simulink model "testemplanner_cs"  (R2020a)
settings: Solver=ode5  StartTime=0.0  StopTime=24  FixedStep=1/1000  RelTol=1e-3
PreLoadFcn:
  | mbxruntime.callbacks.PreLoadFcn(bdroot);
PostLoadFcn:
  | mbxruntime.callbacks.PostLoadFcn(bdroot);
InitFcn:
  | mbxruntime.callbacks.InitFcn(bdroot);
StartFcn:
  | mbxruntime.callbacks.StartFcn(bdroot);
StopFcn:
  | mbxruntime.callbacks.StopFcn(bdroot);
model workspace (MAT data in the model file):
  mbox_table : object (value not decoded)
  model_closed = 0
  sim_status = 0
values from neighbouring files (symbols this model uses):
  c_factor = 43.75    [emplanner_init.m]
  cf = -175016    [emplanner_init.m]
  cr = -130634    [emplanner_init.m]
  global_path_x = [0.057304 1.05668625507 2.05480936558 3.05165624935 4.04722112279 5.04150235808 6.03449985569 7.02621407764 8.01664569183 9.00579544113 9.99366409523 10.9802524329 ... (3001 elements, 3001x1)]    [global_path.mat]
  global_path_y = [8.29 8.29 8.29 8.29 8.29 8.29 8.29 8.29 8.29 8.29 8.29 8.29 ... (3001 elements, 3001x1)]    [global_path.mat]
  KD_PID_distance = 0.0    (= 0)    [emplanner_init.m]
  KD_PID_speed = 0    [emplanner_init.m]
  KI_PID_distance = 0.0    (= 0)    [emplanner_init.m]
  KI_PID_speed = 0    [emplanner_init.m]
  KP_PID_distance = 0.5    [emplanner_init.m]
  KP_PID_speed = 1.8    [emplanner_init.m]
  la = 1.265    [emplanner_init.m]
  lb = 2.947-1.265    (= 1.682)    [emplanner_init.m]
  LQR_K1 = k(:,1)'    [emplanner_init.m]
  LQR_K2 = k(:,2)'    [emplanner_init.m]
  LQR_K3 = k(:,3)'    [emplanner_init.m]
  LQR_K4 = k(:,4)'    [emplanner_init.m]
  m = 2020    [emplanner_init.m]
  rack_displacement = [-39.14 , -37.2 , -35.29 , -33.43 , -31.6 , -29.81 , -28.06 , -26.34 , -24.66 ,      -23.01 , -21.38 , -19.79 , -18.23 , -16.69 , -15.18 , -13.7 , -12.23 , -10.8 , -9.38 , -7.98 ,     -6.61 , -5.25 , -3.91 , -2.59 , -1.29 , 0 , 1.27 , 2.54 , 3.78 , 5.02 , 6.24 , 7.46 , 8.66 ,      9.86 , 11.05 , 12.24 , 13.41 , 14.59 , 15.76 , 16.92 , 18.09 , 19.25 , 20.42 , 21.59 , 22.76 ,      23.93 , 25.11 , 26 ...(+26 chars)    [emplanner_init.m]
  right_wheel_ground = [-70 ,-67.2 , -64.4 , -61.6 , -58.8 , -56 , -53.2 , -50.4 , -47.6 , -44.8 , -42 ,      -39.2 , -36.4 , -33.6 , -30.8 , -28 , -25.2 , -22.4 , -19.6 , -16.8 , -14 , -11.2 , -8.4 , -5.6 ,      -2.8 , 0 , 2.8 , 5.6 , 8.4 , 11.2 , 14 , 16.8 , 19.6 , 22.4 , 25.2 , 28 , 30.8 , 33.6 , 36.4 ,      39.2 , 42 , 44.8 , 47.6 , 50.4 , 53.2 , 56 , 58.8 , 61.6 , 64.4 , 67.2 , 70 ]    [emplanner_init.m]
  vx_break_point = zeros(1,5000)    [emplanner_init.m]
undefined symbols (not defined in the file or in its folder): aubr, DiscIntNeverNeededParam, tablebr, vubr
libraries: PreScanSimulinkLibrary x9, Solver_SF x1, simulink_extras x1
(part 7 of 9)

== matlab function testemplanner_cs/Audi_A8_Sedan_1/decision&planning module/EM Planner/obs1/MATLAB Function2 ==
  data: x_set input; match_point_index_set output; y_set input; frenet_path_x input; frenet_path_y input; frenet_path_heading input; frenet_path_kappa input; proj_x_set output; proj_y_set output; proj_heading_set output; proj_kappa_set output
function [match_point_index_set,proj_x_set, proj_y_set,proj_heading_set,proj_kappa_set] = ...
    fcn(x_set,y_set,frenet_path_x,frenet_path_y,frenet_path_heading,frenet_path_kappa)
%该函数将批量计算x_set，y_set中的xy，在frenet_path下的投影的信息
%输入 x_set,y_set，待投影的点的集合
%x_set,y_set,frenet_path_x,frenet_path_y,frenet_path_heading,frenet_path_kappa
%曲线在直角坐标系下的x，y，heading，kappa
%输出：match_point_index_set 匹配点在frenet_path下的编号的集合(即从全局路径第一个点开始数，第几个点是匹配点)
%     proj_x y heading kappa 投影的x,y,heading,kappa的集合

% 由于事先不知道x_set中到底有多少个点需要投影，因此事先声明一个最大的数量的点作为缓冲
n = 128;
% 并且由于不知道投影点的个数，所以也不知道输出的个数，因此输出也要做缓冲，用nan表示不存在的点
% 输出最多输出128个
% 输出初始化
match_point_index_set = ones(n,1) * nan;
proj_x_set = ones(n,1) * nan;
proj_y_set = ones(n,1) * nan;
proj_heading_set = ones(n,1) * nan;
proj_kappa_set = ones(n,1) * nan;

%找匹配点，需要利用上一个周期的结果作为下一个周期遍历的起点，因此需要声明两个全局变量
persistent is_first_run;
persistent pre_match_point_index_set;
persistent pre_frenet_path_x;
persistent pre_frenet_path_y;
persistent pre_frenet_path_heading;
persistent pre_frenet_path_kappa;
%算法主函数入口

if isempty(is_first_run)
    %该if分支表示函数首次运行
    is_first_run = 0;
    pre_frenet_path_x = frenet_path_x;
    pre_frenet_path_y = frenet_path_y;
    pre_frenet_path_heading = frenet_path_heading;
    pre_frenet_path_kappa = frenet_path_kappa;
    %要记录首次运行计算的匹配点的结果供下个周期运行，先初始化
    pre_match_point_index_set = ones(n,1) * nan;
    %对x_set,y_set的点做遍历，找到他们的匹配点
    for i = 1 : length(x_set)
        if isnan(x_set(i))
            break;
        end
        %首次运行时，没有任何提示，只能从frenet path的第一个点开始找
        start_search_index = 1;
        % 声明increase_count，用于表示在遍历时distance连续增加的个数
        increase_count = 0;
        % 开始遍历
        min_distance = inf;
        for j = start_search_index : length(frenet_path_x)
            distance = (x_set(i) - frenet_path_x(j))^2 + (y_set(i) - frenet_path_y(j))^2;
            if distance < min_distance
                min_distance = distance;
                match_point_index_set(i) = j;
                increase_count = 0;
            else
                increase_count = increase_count + 1;
            end
            %如果distance连续增加50次就不要再遍历了，节省时间
            if increase_count > 50
                break;
            end
        end
        
        %如何通过匹配点计算投影点，请参见《自动驾驶控制算法第七讲》
        %或《自动驾驶决策规划算法》第一章第三节
        
        %取出匹配点的编号
        match_point_index = match_point_index_set(i);
        %取出匹配点的信息
        match_point_x = frenet_path_x(match_point_index);
        match_point_y = frenet_path_y(match_point_index);
        match_point_heading = frenet_path_heading(match_point_index);
        match_point_kappa = frenet_path_kappa(match_point_index);
        %计算匹配点的方向向量与法向量
        vector_match_point = [match_point_x;match_point_y];
        vector_match_point_direction = [cos(match_point_heading);sin(match_point_heading)];
        %声明待投影点的位矢
        vector_r = [x_set(i);y_set(i)];
        
       %通过匹配点计算投影点
       vector_d = vector_r - vector_match_point;
       ds = vector_d' * vector_match_point_direction;
       vector_proj_point = vector_match_point + ds * vector_match_point_direction;
       proj_heading = match_point_heading + match_point_kappa * ds;
       proj_kappa = match_point_kappa;
       %计算结果输出
       proj_x_set(i) = vector_proj_point(1);
       proj_y_set(i) = vector_proj_point(2);
       proj_heading_set(i) = proj_heading;
       proj_kappa_set(i) = proj_kappa;
    end
    %匹配点的计算结果保存，供下一个周期使用
    pre_match_point_index_set = match_point_index_set;
else
    %此if分支表示不是首次运行
    
    %对每个x_set上的点做处理
    for i = 1 : length(x_set)
        %不是首次运行，对于点x_set(i),y_set(i)来说,start_search_index =
        %pre_match_point_index_set(i)
        start_search_index = pre_match_point_index_set(i);%上个周期匹配点的编号作为本周期搜索的起点
        % 声明increase_count，用于表示在遍历时distance连续增加的个数
        %%%%%%%%%
        %对于障碍物检测而言，当感知第一次检测到障碍物时，算法并不是首次运行，此时 
        %pre_match_point_index_set的值是nan，如果还用上一时刻的结果作为本周期搜索的起点
        %必然会出问题，所以要修改
        % 声明increase_count_limit
        increase_count_limit = 5;
        if isnan(start_search_index)
            %没有上个周期的结果，那就不能只检查5次了
            increase_count_limit = 50;
            %搜索起点也要设为1
            start_search_index = 1;
        end
        increase_count = 0;
        % 开始遍历
        %这里多一个步骤，判断遍历的方向
        %计算上个周期匹配点的位矢
        vector_pre_match_point = [pre_frenet_path_x(start_search_index);pre_frenet_path_y(start_search_index)];
        vector_pre_match_point_direction = ...
            [cos(pre_frenet_path_heading(start_search_index));sin(pre_frenet_path_heading(start_search_index))];
        %判断遍历的方向
        flag = ([x_set(i);y_set(i)] - vector_pre_match_point)' * vector_pre_match_point_direction;
        min_distance = inf;
        if flag > 0.001
            for j = start_search_index : length(frenet_path_x)
                distance = (x_set(i) - frenet_path_x(j))^2 + (y_set(i) - frenet_path_y(j))^2;
                if distance < min_distance
                    min_distance = distance;
                    match_point_index_set(i) = j;
                    increase_count = 0;
                else
                    increase_count = increase_count + 1;
                end
                %如果distance连续增加increase_count_limit次就不要再遍历了，节省时间
                if increase_count > increase_count_limit
                    break;
                end
            end
        elseif flag < - 0.001
            for j = start_search_index : -1 : 1
                distance = (x_set(i) - frenet_path_x(j))^2 + (y_set(i) - frenet_path_y(j))^2;
                if distance < min_distance
                    min_distance = distance;
                    match_point_index_set(i) = j;
                    increase_count = 0;
                else
                    increase_count = increase_count + 1;
                end
                %如果distance连续增加increase_count_limit次就不要再遍历了，节省时间
                if increase_count > increase_count_limit
                    break;
                end
            end
        else
            match_point_index_set(i) = start_search_index;
        end
        
        %如何通过匹配点计算投影点，请参见《自动驾驶控制算法第七讲》
        %或《自动驾驶决策规划算法》第一章第三节
        
        %取出匹配点的编号
        match_point_index = match_point_index_set(i);
        %取出匹配点的信息
        match_point_x = frenet_path_x(match_point_index);
        match_point_y = frenet_path_y(match_point_index);
        match_point_heading = frenet_path_heading(match_point_index);
        match_point_kappa = frenet_path_kappa(match_point_index);
        %计算匹配点的方向向量与法向量
        vector_match_point = [match_point_x;match_point_y];
        vector_match_point_direction = [cos(match_point_heading);sin(match_point_heading)];
        %声明待投影点的位矢
        vector_r = [x_set(i);y_set(i)];
        
       %通过匹配点计算投影点
       vector_d = vector_r - vector_match_point;
       ds = vector_d' * vector_match_point_direction;
       vector_proj_point = vector_match_point + ds * vector_match_point_direction;
       proj_heading = match_point_heading + match_point_kappa * ds;
       proj_kappa = match_point_kappa;
       %计算结果输出
       proj_x_set(i) = vector_proj_point(1);
       proj_y_set(i) = vector_proj_point(2);
       proj_heading_set(i) = proj_heading;
       proj_kappa_set(i) = proj_kappa;
  
    end
    %匹配点的计算结果保存，供下一个周期使用
    pre_match_point_index_set = match_point_index_set;
    pre_frenet_path_x = frenet_path_x;
    pre_frenet_path_y = frenet_path_y;
    pre_frenet_path_heading = frenet_path_heading;
    pre_frenet_path_kappa = frenet_path_kappa;
end

== matlab function testemplanner_cs/Audi_A8_Sedan_1/decision&planning module/EM Planner/obs1/obs_fliter ==
  data: host_x input; obs_x_set_gcs_afterfliter output; host_y input; host_heading_xy input; obs_x_set_gcs input; obs_y_set_gcs input; obs_velocity_set_gcs input; obs_heading_set_gcs input; obs_y_set_gcs_afterfliter output; obs_velocity_set_gcs_afterfliter output; obs_heading_set_gcs_afterfliter output
function [obs_x_set_gcs_afterfliter,obs_y_set_gcs_afterfliter,obs_velocity_set_gcs_afterfliter,obs_heading_set_gcs_afterfliter] = fcn(host_x,host_y,host_heading_xy,obs_x_set_gcs,obs_y_set_gcs,obs_velocity_set_gcs,obs_heading_set_gcs)
%%作用：进行障碍筛选，只有在车辆纵向距离为[-10,60],横向距离为[-10，10]的障碍物才被处理
%%输入：车辆的坐标和航向，障碍物的坐标、速度和航向
%%输出：经过筛选后的障碍物的坐标、速度和航向

%%首先做一个缓冲
n=32; %只使用32个障碍物
obs_x_set_gcs_afterfliter=ones(n,1)*nan;
obs_y_set_gcs_afterfliter=ones(n,1)*nan;
obs_velocity_set_gcs_afterfliter=ones(n,1)*nan;
obs_heading_set_gcs_afterfliter=ones(n,1)*nan;
count=1;
%%
for i=1:length(obs_x_set_gcs)
    if isnan(obs_x_set_gcs(i))
        break;
    end
      %先求车辆坐标系的切向量和法向量
%切向量
tor=[cos(host_heading_xy(i));sin(host_heading_xy(i))];
%法向量
nor=[-sin(host_heading_xy(i));cos(host_heading_xy(i))];

lon_distance = [obs_x_set_gcs(i)-host_x;obs_y_set_gcs(i)-host_y]'*tor;
lat_distance = [obs_x_set_gcs(i)-host_x;obs_y_set_gcs(i)-host_y]'*nor;

if lon_distance>=-10 && lon_distance<=60&&lat_distance>=-10 && lat_distance<=10
    obs_x_set_gcs_afterfliter(count)=obs_x_set_gcs(i);
    obs_y_set_gcs_afterfliter(count)=obs_y_set_gcs(i);
    obs_velocity_set_gcs_afterfliter(count)=obs_velocity_set_gcs(i);
    obs_heading_set_gcs_afterfliter(count)=obs_heading_set_gcs(i);
    count=count+1;
end
end

== matlab function testemplanner_cs/Audi_A8_Sedan_1/decision&planning module/EM Planner/DP path1 ==
  data: obs_s_set input; obs_l_set input; plan_start_s input; dp_path_s output; plan_start_l input; plan_start_dl input; plan_start_ddl input; w_collision_cost input; w_smooth_dl_cost input; w_smooth_ddl_cost input; w_smooth_dddl_cost input; w_ref_cost input; row input; col input; sample_s input; sample_l input; dp_path_l output
function [dp_path_s,dp_path_l] = fcnobs_s_set(obs_s_set,obs_l_set,plan_start_s,plan_start_l,plan_start_dl,...
    plan_start_ddl,w_collision_cost,w_smooth_dl_cost,w_smooth_ddl_cost,w_smooth_dddl_cost,w_ref_cost,row,col,sample_s,sample_l)
%%作用：撒点，通过动态规划算出代价最小的路径点集合，算出要进行优化的凸空间
%%输入：规划起点的s，l,dl,ddl,静态障碍物的s，l集合，dl，ddl，dddl平滑代价，参考线代价以及碰撞代价权重
%%行数：为奇数，列数；采样的横向距离以及纵向距离

%%输出：计算得到的路径点s，l初始值

%首先定义一个代价数组，代表从起点到当前i，j点的总代价，均初始化为inf无穷大
node=ones(row,col)*inf;

%再定义一个pre_node,用来表征node的父节点的坐标索引，均初始化为0，0；假设所有节点的父节点均为起点

pre_node=zeros(row,col);
%首先计算第一列的点的cost，调用CalccostFromStart函数进行计算
for i=1:row
%     node(i,1)=CalccostFromStart(plan_start_s,plan_start_l,plan_start_dl,plan_start_ddl,obs_s_set,obs_l_set,w_smooth_dl_cost,w_collision_cost,w_ref_cost,w_smooth_ddl_cost,w_smooth_dddl_cost,i,row,sample_s,sample_l);
 node(i,1) = CalcStartCost(plan_start_s,plan_start_l,plan_start_dl,...
    plan_start_ddl,i,sample_s,sample_l,w_collision_cost,w_smooth_dl_cost,...
    w_smooth_ddl_cost,w_smooth_dddl_cost,w_ref_cost,obs_s_set,obs_l_set,row);
end
%计算从第二列开始的每一列的最小代价值以及其父节点的索引值，调用CalccostFromNeibor函数进行计算
for j=2:col
     for i = 1:row
   
        %遍历前一列的节点
     for k = 1:row
            %计算前一列节点的s l
                [node,pre_node]=CalccostFromNeibor(plan_start_s,node,pre_node,k,j,obs_s_set,obs_l_set,w_smooth_dl_cost,w_collision_cost,w_ref_cost,w_smooth_ddl_cost,w_smooth_dddl_cost,row,sample_s,sample_l);

     end
    end
end
% 找到最后一列中代价最小的节点
min_cost=node(1,end);
index=1;
for i=2:row
    min_cost_temp=node(i,end);
    if min_cost_temp<min_cost
        index=i;
        min_cost=min_cost_temp;
    else
    end
end

%因为不知道有多少个点，所以做一个缓冲
dp_path_s=ones(15,1)* -1;
dp_path_l=ones(15,1)* -1;

temp_node=zeros(col,1);
cur_index = index;
%从最后一个节点开始，反向找到最小代价路径上的所有点，并放入集合中
for i = 1:col
    pre_index=pre_node(cur_index ,end - i + 1);
    temp_node(col - i + 1)=cur_index;
    cur_index=pre_index;
end
%确定路径上点的s，l值
for i=1:col
    dp_path_s(i)=plan_start_s+sample_s*i;
    dp_path_l(i)=sample_l*((row+1)/2-temp_node(i));
end
end
% 
% %函数CalccostFromNeibor，计算从上一列的临近点到这个点的最小cost值和其父节点的行索引
% function [node,pre_node]=CalccostFromNeibor(plan_start_s,node,pre_node,k,j,obs_s_set,obs_l_set,w_smooth_dl_cost,w_collision_cost,w_ref_cost,w_smooth_ddl_cost,w_smooth_dddl_cost,row,sample_s,sample_l)
% % %作用： 计算从从上一列的临近点到这个点的最小cost值和其父节点的行索引
%   %输入：起点的s，l，障碍物的s,l,dl,ddl,dddl平滑权重，障碍物碰撞权重，参考线权重，当前所在行数，列数，总行数，采样s，l，node和pre_node数组
%   %输出：更新后的node和pre_node数组
%   %dl，ddl设为0，因为DP仅仅是为了粗略开辟凸空间，不用太精细。
% start_s=plan_start_s+sample_s*(j-1);
% end_s=start_s+sample_s;
% start_dl=0;
% start_ddl=0;
% end_dl=0;
% end_ddl=0;
% cost=zeros(row,1);
% %确定起点和终点参数，计算五次多项式系数
% for i=1:row
% start_l=sample_l*((row+1)/2-i);
% end_l=sample_l*((row+1)/2-k);
% %调用函数计算五次多项式系数
% coffee=CalcQuinticCoeffient(start_l,start_dl,start_ddl,end_l,end_dl,end_ddl,start_s,end_s);
% 
% s_set=zeros(10,1);
% l_set=zeros(10,1);
% dl_set=zeros(10,1);
% ddl_set=zeros(10,1);
% dddl_set=zeros(10,1);
% 
% %找10个点进行代价计算
% for n=1:10
%     s_set(n)=start_s+sample_s/10*(n-1);
%     l_set(n)=coffee(6)*(s_set(n))^5+coffee(5)*(s_set(n))^4+coffee(4)*(s_set(n))^3+coffee(3)*(s_set(n))^2+coffee(2)*(s_set(n))+coffee(1);
%     dl_set(n)=5*coffee(6)*(s_set(n))^4+4*coffee(5)*(s_set(n))^3+3*coffee(4)*(s_set(n))^2+2*coffee(3)*(s_set(n))+coffee(2);
%     ddl_set(n)=20*coffee(6)*(s_set(n))^3+12*coffee(5)*(s_set(n))^2+6*coffee(4)*(s_set(n))+2*coffee(3);
%     dddl_set(n)=60*coffee(6)*(s_set(n))^2+24*coffee(5)*(s_set(n))+6*coffee(4);
% end
% %首先计算平滑带代价和参考线代价
% smooth_cost=w_smooth_dl_cost*(dl_set'*dl_set)+w_smooth_ddl_cost*(ddl_set'*ddl_set)+w_smooth_dddl_cost*(dddl_set'*dddl_set);
% ref_cost=w_ref_cost*(l_set'*l_set);
% %接着计算障碍物代价
% collision_cost=0;
% for m=1:length(obs_s_set)
%     if isnan(obs_s_set(m))
%         break;
%     end
%     s_err=obs_s_set(m)*ones(10,1)-s_set;
%     l_err=obs_l_set(m)*ones(10,1)-l_set;
%     err_squard=s_err.^2+l_err.^2;
%     %调用障碍物代价模型函数CalcObsCost进行计算
%     collision_cost_one=CalcObsCost(w_collision_cost,err_squard);
%     collision_cost=collision_cost+collision_cost_one;
% end
% 
% cost(i)=smooth_cost+ref_cost+collision_cost+node(i,j-1);
% end
% index=1;
% min_cost=cost(1);
% for h =2:row
%    
%     min_cost_temp=cost(h);
%     if min_cost_temp<min_cost
%         index=h;
%         min_cost=min_cost_temp;
%     else
%     end
% end
%  pre_node(k,j)=index;
%  node(k,j)=min_cost;
% end
% 
% 
% 
% % %函数CalccostFromStart，计算从起点到第一列的点的cost值
% function cost=CalcStartCost(plan_start_s,plan_start_l,plan_start_dl,plan_start_ddl,node_row,sample_s,sample_l,w_collision_cost,w_smooth_dl_cost,w_smooth_ddl_cost,w_smooth_dddl_cost,w_ref_cost,obs_s_set,obs_l_set,row)
% 
%   %作用： 计算从起点到第一列的点的cost值
%   %输入：起点的s，l，dl，ddl,障碍物的s,l,dl,ddl,dddl平滑权重，障碍物碰撞权重，参考线权重，当前所在行数，总行数，采样s，l
%   %输出：代价和
% start_s=plan_start_s;
% start_l=plan_start_l;
% start_dl=plan_start_dl;
% start_ddl=plan_start_ddl;
% end_s=start_s+sample_s;
% end_l=sample_l*((row+1)/2-node_row);
% end_dl=0;
% end_ddl=0;
% %调用函数计算五次多项式系数
% coffee=CalcQuinticCoeffient(start_l,start_dl,start_ddl,end_l,end_dl,end_ddl,start_s,end_s);
% 
% s_set=zeros(10,1);
% l_set=zeros(10,1);
% dl_set=zeros(10,1);
% ddl_set=zeros(10,1);
% dddl_set=zeros(10,1);
% 
% %找10个点进行代价计算
% for i=1:10
%     s_set(i)=start_s+sample_s/10*(i-1);
%     l_set(i)=coffee(6)*(s_set(i))^5+coffee(5)*(s_set(i))^4+coffee(4)*(s_set(i))^3+coffee(3)*(s_set(i))^2+coffee(2)*(s_set(i))+coffee(1);
%     dl_set(i)=5*coffee(6)*(s_set(i))^4+4*coffee(5)*(s_set(i))^3+3*coffee(4)*(s_set(i))^2+2*coffee(3)*(s_set(i))+coffee(2);
%     ddl_set(i)=20*coffee(6)*(s_set(i))^3+12*coffee(5)*(s_set(i))^2+6*coffee(4)*(s_set(i))+2*coffee(3);
%     dddl_set(i)=60*coffee(6)*(s_set(i))^2+24*coffee(5)*(s_set(i))+6*coffee(4);
% end
% %首先计算平滑带代价和参考线代价
% smooth_cost=w_smooth_dl_cost*(dl_set'*dl_set)+w_smooth_ddl_cost*(ddl_set'*ddl_set)+w_smooth_dddl_cost*(dddl_set'*dddl_set);
% ref_cost=w_ref_cost*(l_set'*l_set);
% %接着计算障碍物代价
% collision_cost=0;
% for i=1:length(obs_s_set)
%     if isnan(obs_s_set(i))
%         break;
%     end
%     s_err=obs_s_set(i)*ones(10,1)-s_set;
%     l_err=obs_l_set(i)*ones(10,1)-l_set;
%     err_squard=s_err.^2+l_err.^2;
%      %调用障碍物代价模型函数CalcObsCost进行计算
%     collision_cost_one=CalcObsCost(w_collision_cost,err_squard);
%     collision_cost=collision_cost+collision_cost_one;
% end
% 
% cost=smooth_cost+ref_cost+collision_cost;
% 
% 
% end
% 
% 
% 
% function coffee=CalcQuinticCoeffient(start_l,start_dl,start_ddl,end_l,end_dl,end_ddl,start_s,end_s)
%   %作用：计算五次多项式系数
%   %输入：起点和终点的s,l,dl,ddl共6个值
%   %输出：六个权重系数
%     start_s2=start_s*start_s;
%     start_s3=start_s2*start_s;
%     start_s4=start_s3*start_s;
%     start_s5=start_s4*start_s;
%     end_s2=end_s*end_s;
%     end_s3=end_s2*end_s;
%     end_s4=end_s3*end_s;
%     end_s5=end_s4*end_s;
%     A=[1,start_s,start_s2,start_s3,start_s4,start_s5;
%        0,1,2*start_s,3*start_s2,4*start_s3,5*start_s4;
%        0,0,2,6*start_s,12*start_s2,20*start_s3;
%        1,end_s,end_s2,end_s3,end_s4,end_s5;
%        0,1,2*end_s,3*end_s2,4*end_s3,5*end_s4;
%         0,0,2,6*end_s,12*end_s2,20*end_s3;];
%     B=[start_l;start_dl;start_ddl;end_l;end_dl;end_ddl];
%     coffee=A\B;
% end
% 
% 
% % function obscost=CalcObsCost(w_collision_cost,err_squard)
% %   %作用： %建立一个障碍物评估模型，进行代价评估
% %   %输入：与障碍物的横纵向距离平方和，碰撞权重
% %   %输出：障碍物代价和
% %     cost=0;
% %     for i=1:length(err_squard)
% %         
% %         if (err_squard(i)<16 )&&(err_squard(i)>9)
% %             cost=cost+1000/err_squard(i);
% %         elseif (err_squard(i)<9 )
% %             cost=cost+w_collision_cost;
% %         end
% %     end
% %     obscost=cost;
% % end
% function obs_cost = CalcObsCost(w_cost_collision,square_d)
% %该函数将计算障碍物的距离代价
% % 暂定超过4米的cost为0 在4到3米的cost为1000/squard_d,在小于3米的cost为w_cost_collision
%   cost = 0;
%   for i = 1:length(square_d)
%       if (square_d(i) < 16) && (square_d(i) > 9) 
%           cost = cost + 1000/square_d(i);
%       elseif (square_d(i) < 9)
%           cost = cost + w_cost_collision;
%       end
%   end
%   obs_cost = cost;
% 
% end

function [node,pre_node]=CalccostFromNeibor(plan_start_s,node,pre_node,k,j,obs_s_set,obs_l_set,w_smooth_dl_cost,w_collision_cost,w_ref_cost,w_smooth_ddl_cost,w_smooth_dddl_cost,row,sample_s,sample_l)
% %作用： 计算从从上一列的临近点到这个点的最小cost值和其父节点的行索引
  %输入：起点的s，l，障碍物的s,l,dl,ddl,dddl平滑权重，障碍物碰撞权重，参考线权重，当前所在行数，列数，总行数，采样s，l，node和pre_node数组
  %输出：更新后的node和pre_node数组
  %dl，ddl设为0，因为DP仅仅是为了粗略开辟凸空间，不用太精细。
start_s=plan_start_s+sample_s*(j-1);
end_s=start_s+sample_s;
start_dl=0;
start_ddl=0;
end_dl=0;
end_ddl=0;
cost=zeros(row,1);
%确定起点和终点参数，计算五次多项式系数
for i=1:row
start_l=sample_l*((row+1)/2-i);
end_l=sample_l*((row+1)/2-k);
%调用函数计算五次多项式系数
coffee=CalcQuinticCoeffient(start_l,start_dl,start_ddl,end_l,end_dl,end_ddl,start_s,end_s);

s_set=zeros(10,1);
l_set=zeros(10,1);
dl_set=zeros(10,1);
ddl_set=zeros(10,1);
dddl_set=zeros(10,1);

%找10个点进行代价计算
for n=1:10
    s_set(n)=start_s+sample_s/10*(n-1);
    l_set(n)=coffee(6)*(s_set(n))^5+coffee(5)*(s_set(n))^4+coffee(4)*(s_set(n))^3+coffee(3)*(s_set(n))^2+coffee(2)*(s_set(n))+coffee(1);
    dl_set(n)=5*coffee(6)*(s_set(n))^4+4*coffee(5)*(s_set(n))^3+3*coffee(4)*(s_set(n))^2+2*coffee(3)*(s_set(n))+coffee(2);
    ddl_set(n)=20*coffee(6)*(s_set(n))^3+12*coffee(5)*(s_set(n))^2+6*coffee(4)*(s_set(n))+2*coffee(3);
    dddl_set(n)=60*coffee(6)*(s_set(n))^2+24*coffee(5)*(s_set(n))+6*coffee(4);
end
%首先计算平滑带代价和参考线代价
smooth_cost=w_smooth_dl_cost*(dl_set'*dl_set)+w_smooth_ddl_cost*(ddl_set'*ddl_set)+w_smooth_dddl_cost*(dddl_set'*dddl_set);
ref_cost=w_ref_cost*(l_set'*l_set);
%接着计算障碍物代价
collision_cost=0;
for m=1:length(obs_s_set)
    if isnan(obs_s_set(m))
        break;
    end
    s_err=obs_s_set(m)*ones(10,1)-s_set;
    l_err=obs_l_set(m)*ones(10,1)-l_set;
    err_squard=s_err.^2+l_err.^2;
    %调用障碍物代价模型函数CalcObsCost进行计算
    collision_cost_one=CalcObsCost(w_collision_cost,err_squard);
    collision_cost=collision_cost+collision_cost_one;
end

cost(i)=smooth_cost+ref_cost+collision_cost+node(i,j-1);
end
index=1;
min_cost=cost(1);
for h =2:row
   
    min_cost_temp=cost(h);
    if min_cost_temp<min_cost
        index=h;
        min_cost=min_cost_temp;
    else
    end
end
 pre_node(k,j)=index;
 node(k,j)=min_cost;
end


function cost=CalcStartCost(plan_start_s,plan_start_l,plan_start_dl,plan_start_ddl,node_row,sample_s,sample_l,w_collision_cost,w_smooth_dl_cost,w_smooth_ddl_cost,w_smooth_dddl_cost,w_ref_cost,obs_s_set,obs_l_set,row)

  %作用： 计算从起点到第一列的点的cost值
  %输入：起点的s，l，dl，ddl,障碍物的s,l,dl,ddl,dddl平滑权重，障碍物碰撞权重，参考线权重，当前所在行数，总行数，采样s，l
  %输出：代价和
start_s=plan_start_s;
start_l=plan_start_l;
start_dl=plan_start_dl;
start_ddl=plan_start_ddl;
end_s=start_s+sample_s;
end_l=sample_l*((row+1)/2-node_row);
end_dl=0;
end_ddl=0;
%调用函数计算五次多项式系数
coffee=CalcQuinticCoeffient(start_l,start_dl,start_ddl,end_l,end_dl,end_ddl,start_s,end_s);

s_set=zeros(10,1);
l_set=zeros(10,1);
dl_set=zeros(10,1);
ddl_set=zeros(10,1);
dddl_set=zeros(10,1);

%找10个点进行代价计算
for i=1:10
    s_set(i)=start_s+sample_s/10*(i-1);
    l_set(i)=coffee(6)*(s_set(i))^5+coffee(5)*(s_set(i))^4+coffee(4)*(s_set(i))^3+coffee(3)*(s_set(i))^2+coffee(2)*(s_set(i))+coffee(1);
    dl_set(i)=5*coffee(6)*(s_set(i))^4+4*coffee(5)*(s_set(i))^3+3*coffee(4)*(s_set(i))^2+2*coffee(3)*(s_set(i))+coffee(2);
    ddl_set(i)=20*coffee(6)*(s_set(i))^3+12*coffee(5)*(s_set(i))^2+6*coffee(4)*(s_set(i))+2*coffee(3);
    dddl_set(i)=60*coffee(6)*(s_set(i))^2+24*coffee(5)*(s_set(i))+6*coffee(4);
end
%首先计算平滑带代价和参考线代价
smooth_cost=w_smooth_dl_cost*(dl_set'*dl_set)+w_smooth_ddl_cost*(ddl_set'*ddl_set)+w_smooth_dddl_cost*(dddl_set'*dddl_set);
ref_cost=w_ref_cost*(l_set'*l_set);
%接着计算障碍物代价
collision_cost=0;
for i=1:length(obs_s_set)
    if isnan(obs_s_set(i))
        break;
    end
    s_err=obs_s_set(i)*ones(10,1)-s_set;
    l_err=obs_l_set(i)*ones(10,1)-l_set;
    err_squard=s_err.^2+l_err.^2;
     %调用障碍物代价模型函数CalcObsCost进行计算
    collision_cost_one=CalcObsCost(w_collision_cost,err_squard);
    collision_cost=collision_cost+collision_cost_one;
end

cost=smooth_cost+ref_cost+collision_cost;


end

function obs_cost = CalcObsCost(w_cost_collision,square_d)
%该函数将计算障碍物的距离代价
% 暂定超过4米的cost为0 在4到3米的cost为1000/squard_d,在小于3米的cost为w_cost_collision
  cost = 0;
  for i = 1:length(square_d)
      if (square_d(i) < 16) && (square_d(i) > 9) 
          cost = cost + 1000/square_d(i);
      elseif (square_d(i) < 9)
          cost = cost + w_cost_collision;
      end
  end
  obs_cost = cost;

end



function coffee=CalcQuinticCoeffient(start_l,start_dl,start_ddl,end_l,end_dl,end_ddl,start_s,end_s)
  %作用：计算五次多项式系数
  %输入：起点和终点的s,l,dl,ddl共6个值
  %输出：六个权重系数
    start_s2=start_s*start_s;
    start_s3=start_s2*start_s;
    start_s4=start_s3*start_s;
    start_s5=start_s4*start_s;
    end_s2=end_s*end_s;
    end_s3=end_s2*end_s;
    end_s4=end_s3*end_s;
    end_s5=end_s4*end_s;
    A=[1,start_s,start_s2,start_s3,start_s4,start_s5;
       0,1,2*start_s,3*start_s2,4*start_s3,5*start_s4;
       0,0,2,6*start_s,12*start_s2,20*start_s3;
       1,end_s,end_s2,end_s3,end_s4,end_s5;
       0,1,2*end_s,3*end_s2,4*end_s3,5*end_s4;
        0,0,2,6*end_s,12*end_s2,20*end_s3;];
    B=[start_l;start_dl;start_ddl;end_l;end_dl;end_ddl];
    coffee=A\B;
end

== matlab function testemplanner_cs/Audi_A8_Sedan_1/decision&planning module/EM Planner/obs1/obs_fliter_for_static ==
  data: obs_x_set_gcs_afterfliter input; obs_x_set_gcs_static output; obs_y_set_gcs_afterfliter input; obs_velocity_set_gcs_afterfliter input; obs_heading_set_gcs_afterfliter input; obs_y_set_gcs_static output; obs_x_set_gcs_dynamic output; obs_y_set_gcs_dynamic output; obs_vx_set_gcs_dynamic output; obs_vy_set_gcs_dynamic output
function [obs_x_set_gcs_static,obs_y_set_gcs_static,obs_x_set_gcs_dynamic,obs_y_set_gcs_dynamic,obs_vx_set_gcs_dynamic,obs_vy_set_gcs_dynamic] = fcn(obs_x_set_gcs_afterfliter,obs_y_set_gcs_afterfliter,obs_velocity_set_gcs_afterfliter,obs_heading_set_gcs_afterfliter)
%%作用：进行障碍筛选，只有在车辆纵向距离为[-10,60],横向距离为[-10，10]的障碍物才被处理
%%输入：车辆的坐标和航向，障碍物的坐标、速度和航向
%%输出：经过筛选后的障碍物的坐标、速度和航向

%%首先做一个缓冲
n=32; %只使用32个障碍物
obs_x_set_gcs_static=ones(n,1)*nan;
obs_y_set_gcs_static=ones(n,1)*nan;
obs_x_set_gcs_dynamic=ones(n,1)*nan;
obs_y_set_gcs_dynamic=ones(n,1)*nan;
obs_vx_set_gcs_dynamic=ones(n,1)*nan;
obs_vy_set_gcs_dynamic=ones(n,1)*nan;
count_static=1;
count_dynamic=1;
%%
for i=1:length(obs_x_set_gcs_afterfliter)
   
if abs(obs_velocity_set_gcs_afterfliter(i))<0.1
    obs_x_set_gcs_static(count_static)=obs_x_set_gcs_afterfliter(i);
    obs_y_set_gcs_static(count_static)=obs_y_set_gcs_afterfliter(i);
    count_static=count_static+1;
else
    obs_x_set_gcs_dynamic(count_dynamic)=obs_x_set_gcs_afterfliter(i);
    obs_y_set_gcs_dynamic(count_dynamic)=obs_y_set_gcs_afterfliter(i);
    obs_vx_set_gcs_dynamic(count_dynamic)=obs_velocity_set_gcs_afterfliter(i)*cos(obs_heading_set_gcs_afterfliter(i));
    obs_vy_set_gcs_dynamic(count_dynamic)=obs_velocity_set_gcs_afterfliter(i)*sin(obs_heading_set_gcs_afterfliter(i));
    count_dynamic=count_dynamic+1;
end
end

== matlab function testemplanner_cs/Audi_A8_Sedan_1/decision&planning module/EM Planner/obs1/obs filter1 ==
  data: host_x input; obs_x_set_final output; host_y input; host_heading_xy input; obs_x_set_gcs input; obs_y_set_gcs input; obs_velocity_set_gcs input; obs_heading_set_gcs input; obs_y_set_final output; obs_velocity_set_final output; obs_heading_set_final output
function [obs_x_set_final,obs_y_set_final,obs_velocity_set_final,obs_heading_set_final] = fcn(host_x,host_y,host_heading_xy,obs_x_set_gcs,obs_y_set_gcs,obs_velocity_set_gcs,obs_heading_set_gcs)
% 该函数将筛选障碍物，纵向[-10,60] 横向[-10,10]的障碍物才会被考虑
% 该函数只是一种单车道的临时办法，考虑到多车道情况，即使障碍物距离较远也应该考虑
% EM Planner完全体是多车道并行计算的，每个车道都生成参考线然后并行计算出多条轨迹，再选择最优的轨迹作为输出

%传感器最多可以识别32个障碍物
n = 32;
%输出初始化
obs_x_set_final = ones(n,1)*nan;
obs_y_set_final = ones(n,1)*nan;
obs_velocity_set_final = ones(n,1)*nan;
obs_heading_set_final = ones(n,1)*nan;
count = 1;
for i = 1:length(obs_x_set_gcs)
    if isnan(obs_x_set_gcs(i))
        break;
    end
    %自车的heading的方向向量与法向量
    tor = [cos(host_heading_xy);sin(host_heading_xy)];
    nor = [-sin(host_heading_xy);cos(host_heading_xy)];
    %障碍物与自车的距离向量
    vector_obs = [obs_x_set_gcs(i);obs_y_set_gcs(i)] - [host_x;host_y];
    %障碍物纵向距离
    lon_distance = vector_obs'*tor;
    %障碍物横向距离
    lat_distance = vector_obs'*nor;
    
    if (lon_distance < 60) && (lon_distance > -10) && (lat_distance > -10) && (lat_distance < 10)
        obs_x_set_final(count) = obs_x_set_gcs(i);
        obs_y_set_final(count) = obs_y_set_gcs(i);
        obs_heading_set_final(count) = obs_heading_set_gcs(i);
        obs_velocity_set_final(count) = obs_velocity_set_gcs(i);
        count = count + 1;
    end
end

== matlab function testemplanner_cs/Audi_A8_Sedan_1/decision&planning module/EM Planner/obs1/MATLAB Function1 ==
  data: obs_x_set_gcs input; static_obs_x_set output; obs_y_set_gcs input; obs_heading_set_gcs input; obs_velocity_set_gcs input; static_obs_y_set output; dynamic_obs_x_set output; dynamic_obs_y_set output; dynamic_obs_vx_set output; dynamic_obs_vy_set output
function [static_obs_x_set,static_obs_y_set,dynamic_obs_x_set,dynamic_obs_y_set,dynamic_obs_vx_set,dynamic_obs_vy_set]...
    = fcn(obs_x_set_gcs,obs_y_set_gcs,obs_heading_set_gcs,obs_velocity_set_gcs)

%该函数将分类静态障碍物和动态障碍物
%输出初始化
n = 32;
static_obs_x_set = ones(n,1)*nan;
static_obs_y_set = ones(n,1)*nan;
dynamic_obs_x_set = ones(n,1)*nan;
dynamic_obs_y_set = ones(n,1)*nan;
dynamic_obs_vx_set = ones(n,1)*nan;
dynamic_obs_vy_set = ones(n,1)*nan;
count_static = 1;
count_dynamic = 1;
for i = 1:length(obs_x_set_gcs)
    if abs(obs_velocity_set_gcs(i)) < 0.1
        static_obs_x_set(count_static) = obs_x_set_gcs(i);
        static_obs_y_set(count_static) = obs_y_set_gcs(i);
        count_static = count_static + 1;
    else
        dynamic_obs_x_set(count_dynamic) = obs_x_set_gcs(i);
        dynamic_obs_y_set(count_dynamic) = obs_y_set_gcs(i);
        dynamic_obs_vx_set(count_dynamic) = obs_velocity_set_gcs(i)*cos(obs_heading_set_gcs(i));
        dynamic_obs_vy_set(count_dynamic) = obs_velocity_set_gcs(i)*sin(obs_heading_set_gcs(i));
        count_dynamic = count_dynamic + 1;      
    end
end

== matlab function testemplanner_cs/Audi_A8_Sedan_1/control module3/MATLAB Function ==
  data: trajectory_x input; xr output; trajectory_y input; trajectory_heading input; trajectory_kappa input; trajectory_speed input; trajectory_accel input; trajectory_time input; current_time input; yr output; thetar output; kappar output; vr output; ar output
function [xr,yr,thetar,kappar,vr,ar] = fcn(trajectory_x,trajectory_y,trajectory_heading,...
    trajectory_kappa,trajectory_speed,trajectory_accel,trajectory_time,current_time)
% 该函数根据规划的轨迹计算出期望跟踪的点
% 由于控制也是有延迟，所以控制发出的期望跟踪的点是current_time + 0.01;
control_time = current_time + 0.01;
% 规划发出的轨迹有一部分是拼接的，在刚启动的时候，stitch_time = -1,因此要先把它去掉
start_index = 1;
while (trajectory_time(start_index) == -1)
    start_index = start_index + 1;
end
% 使用interp1插值计算得到xr yr thetar,kappar,vr,ar
% 由于interp1在端点会得到nan，因此需要防一手
% 解释，为什么需要trajectory_time(start_index) ~= 0
% 因为在刚启动时规划先执行(100ms)，当规划完毕的时候控制已经执行了10次
% 那么在最开始的时候，规划还没给结果是控制已经执行了10次，在这10次中控制跟踪的轨迹是空轨迹
% simulink 空轨迹表示为 0，0，0，0，0，0......,这样trajectory_time
% 也全是0，trajectory_time不单调递增
% 而interp1(x,y,x0)要求x必须要单调递增，否则会报错，所以当规划首次运行时控制需要执行下面这个else分支的代码，否则会报错
if control_time > trajectory_time(start_index) && trajectory_time(start_index) ~= 0
    xr = interp1(trajectory_time(start_index:end),trajectory_x(start_index:end),control_time);
    yr = interp1(trajectory_time(start_index:end),trajectory_y(start_index:end),control_time);
    thetar = interp1(trajectory_time(start_index:end),trajectory_heading(start_index:end),control_time);
    kappar = interp1(trajectory_time(start_index:end),trajectory_kappa(start_index:end),control_time);
    vr = interp1(trajectory_time(start_index:end),trajectory_speed(start_index:end),control_time);
    ar = interp1(trajectory_time(start_index:end),trajectory_accel(start_index:end),control_time);
else
    xr = trajectory_x(start_index);
    yr = trajectory_y(start_index);
    thetar = trajectory_heading(start_index);
    kappar = trajectory_kappa(start_index);
    vr = trajectory_speed(start_index);
    ar = trajectory_accel(start_index);
end

== stateflow chart testemplanner_cs/Audi_A8_Sedan_1/Schedule OS ==
  (default) -> (junction 5)
  (junction 5) -> (junction 9) [order 1] : [i>100]
  (junction 5) -> (junction 10) [order 2] : {i = i+1;}
  (junction 9) -> (junction 12) : {
      | do_planning;
      | i = 0;
      | }
  (junction 12) -> (junction 10)
  (junction 10) -> (junction 15)
  (junction 15) -> (junction 17) [order 1] : [j>10]
  (junction 15) -> (junction 21) [order 2] : {j = j+1}
  (junction 17) -> (junction 19) : {
      | do_control;
      | j = 0;
      | }
  (junction 19) -> (junction 21)
  (junction 21) -> (junction 24)
  data: i local =1; j local =1
  events: do_planning output FUNCTION_CALL_EVENT; do_control output FUNCTION_CALL_EVENT

== matlab function testemplanner_cs/Audi_A8_Sedan_1/control module2/MATLAB Function2 ==
  data: trajectory_x_final input; x_r output; trajectory_y_final input; trajectory_heading_final input; trajectory_kappa_final input; trajectory_speed_final input; trajectory_accel_final input; trajectory_time_final input; current_time input; y_r output; theta_r output; kappa_r output; speed output; accel output
function [x_r,y_r,theta_r,kappa_r,speed,accel] = fcn(trajectory_x_final,trajectory_y_final,trajectory_heading_final,trajectory_kappa_final,trajectory_speed_final,...
    trajectory_accel_final,trajectory_time_final,current_time)

%%作用，根据当前时间，选取轨迹点集合上合适的点进行插值，生成控制用的x，y,heading,kappa,speed,acc

%%输入：轨迹点集合的x，y,heading,kappa,acc,时间戳，当前时间。

%%输出：控制点用的x，y,heading,kappa,speed,acc


%首先控制也要进行预瞄,时间是0.01/0.02
control_time=current_time+0.01;
start_index=1;
%%为了防止轨迹所对应的时间戳不可信（时间戳为-1），找到可用的起点
while trajectory_time_final(start_index)==-1
        start_index=start_index+1;
end

%%正常来讲可以通过插值的方式（调用matlab函数interp1）来计算控制点对应的插值
%%但是存在着两种异常工况需要进行处理
%%①interp1在段点插值会得到nan
%%②interp1要求x轴的数必须单调递增

%%在起步时：在t=0~100ms时刻，规划还未完成，无轨迹信息，也就是说轨迹的时间都是0，而控制每10ms执行异常，因此此时给控制的轨迹信息应该全为起点的信息
%%保证车辆不动

if trajectory_time_final(start_index)~=0 &&control_time>trajectory_time_final(start_index) %%正常运行分支
    x_r=interp1(trajectory_x_final(start_index:end),trajectory_time_final(start_index:end),control_time);
    y_r=interp1(trajectory_y_final(start_index:end),trajectory_time_final(start_index:end),control_time);
    theta_r=interp1(trajectory_heading_final(start_index:end),trajectory_time_final(start_index:end),control_time);
    if theta_r==-pi
        theta_r=pi;
    elseif theta_r==2*pi||theta_r==-2*pi
        theta_r=0;
    else
    end
    
    kappa_r=interp1(trajectory_kappa_final(start_index:end),trajectory_time_final(start_index:end),control_time);
    speed=interp1(trajectory_speed_final(start_index:end),trajectory_time_final(start_index:end),control_time);
    accel=interp1(trajectory_accel_final(start_index:end),trajectory_time_final(start_index:end),control_time);
else
    
    x_r=trajectory_x_final(start_index);
    y_r=trajectory_y_final(start_index);
    theta_r=trajectory_heading_final(start_index);
    kappa_r=trajectory_kappa_final(start_index);
    speed=trajectory_speed_final(start_index);
    accel=trajectory_accel_final(start_index);

end

end

== matlab function testemplanner_cs/Audi_A8_Sedan_1/control module2/control main/chassic steering system/MATLAB Function ==
  data: u input; right_steer output; la input; lb input
function right_steer = fcn(u,la,lb)
if abs(u)<1e-2
   right_steer = u;
else
   R =  (la+lb)/tan(u);
   right_steer = atan((la+lb)/(R+1.624/2));
end

== matlab function testemplanner_cs/Audi_A8_Sedan_1/control module2/control main/lateral control LQR/calc lqr K ==
  data: k1 input; k output; k2 input; k3 input; k4 input; vx input
function k  = fcn(k1,k2,k3,k4,vx)
    if abs(vx)<0.1
        k=[0,0,0,0];
    else
       
        k=[k1,k2,k3,k4];
    end
end

== matlab function testemplanner_cs/Audi_A8_Sedan_1/control module2/control main/lateral control LQR/err_kappa_calculate_module ==
  data: x input; y input; phi input; vx input; vy input; phi_dot input; xr input; yr input; thetar input; kappar input; err output; es output; s_dot output; phi output; projection_point_thetar output
function [err,es,s_dot,phi,projection_point_thetar] = fcn(x,y,phi,vx,vy,phi_dot,xr,yr,thetar,kappar)
    
    tor=[cos(thetar);sin(thetar)];
    nor=[-sin(thetar);cos(thetar)];
    d_err=[x-xr;y-yr];
    ed=nor'*d_err;
    es=tor'*d_err;
    %projection_point_thetar=thetar(dmin);%apollo
    projection_point_thetar=thetar+kappar*es;
    ed_dot=vy*cos(phi-projection_point_thetar)+vx*sin(phi-projection_point_thetar);
    %%%%%%%%%
    ephi=sin(phi-projection_point_thetar);
    %%%%%%%%%
    ss_dot=vx*cos(phi-projection_point_thetar)-vy*sin(phi-projection_point_thetar);
    s_dot=ss_dot/(1-kappar*ed);
    ephi_dot=phi_dot-kappar*s_dot;
    err=[ed;ed_dot;ephi;ephi_dot];
    
    
    
    
    
    
    
    
    
    
    
    


end

== matlab function testemplanner_cs/Audi_A8_Sedan_1/control module2/control main/lateral control LQR/feed_forword_control ==
  data: vx input; a input; forword_angle output; b input; m input; cf input; cr input; k input; kr input
function forword_angle = fcn(vx,a,b,m,cf,cr,k,kr)
    forword_angle=kr*(a+b-b*k(3)-(m*vx*vx/(a+b))*((b/cf)+(a/cr)*k(3)-(a/cr)));
end

== matlab function testemplanner_cs/Audi_A8_Sedan_1/control module2/control main/lateral control LQR/feedback_control+feedforword_control ==
  data: k input; angle output; err input; forword_angle input
function angle = fcn(k,err,forword_angle)

    angle=-k*err+forword_angle;
end

== matlab function testemplanner_cs/Audi_A8_Sedan_1/control module2/control main/lateral control LQR/predict_module ==
  data: x input; pred_x_ctrl output; y input; phi input; vx input; vy input; phi_dot input; ts input; pred_y_ctrl output; pred_yaw_ctrl output; pred_vx_ctrl output; pred_vy_ctrl output; pred_yaw_dot_ctrl output
function [pred_x_ctrl,pred_y_ctrl,pred_yaw_ctrl,pred_vx_ctrl,pred_vy_ctrl,pred_yaw_dot_ctrl] = fcn(x,y,phi,vx,vy,phi_dot,ts)
    pred_x_ctrl=x+vx*ts*cos(phi)-vy*ts*sin(phi);
    pred_y_ctrl=y+vy*ts*cos(phi)+vx*ts*sin(phi);
    pred_yaw_ctrl=phi;
    pred_vx_ctrl=vx;
    pred_vy_ctrl=vy;
    pred_yaw_dot_ctrl=phi_dot;
end

== matlab function testemplanner_cs/Audi_A8_Sedan_1/control module2/control main/longitudinal control double PID/MATLAB Function1 ==
  data: u input; throttle output; brake output
function [throttle,brake] = fcn(u)
    if u>=0
        throttle=u;
        brake=0;
    else
        throttle=0;
        brake=-u;
    end

== matlab function testemplanner_cs/Audi_A8_Sedan_1/control module3/control main/chassic steering system/MATLAB Function ==
  data: u input; right_steer output; la input; lb input
function right_steer = fcn(u,la,lb)
if abs(u)<1e-2
   right_steer = u;
else
   R =  (la+lb)/tan(u);
   right_steer = atan((la+lb)/(R+1.624/2));
end

== matlab function testemplanner_cs/Audi_A8_Sedan_1/Perciption/Perception Model ==
  data: host_x input; obs_x_set_gcs output; host_y input; host_heading_xy input; obs_range input; obs_theta input; obs_velocity input; obs_heading input; obs_y_set_gcs output; obs_velocity_set_gcs output; obs_heading_set_gcs output
function [obs_x_set_gcs,obs_y_set_gcs,obs_velocity_set_gcs,obs_heading_set_gcs] = fcn(host_x,host_y,host_heading_xy,obs_range,obs_theta,obs_velocity,obs_heading)

%作用：处理传感器所得到的障碍物信息，将其转换为世界坐标系下的障碍物信息。AIR传感器探测到的障碍物速度为世界坐标系下的绝对速度，距离为车辆坐标系下的相对距离，而航向则是以正北为正方向，顺时针为正，
%世界坐标系则是以正东为正方向，逆时针为正，因此需要进行变换(Heading [degs]: Compass heading of the target detected (driving direction where N = 0 degs, E = 90 degs, S = 180 degs and W = 270 degs))
%输入：车辆当前x,y位置和航向
%输出：障碍物在世界坐标系下的x,y位置、速度和航向     
obs_x_set_gcs=ones(32,1)*nan;
obs_y_set_gcs=ones(32,1)*nan;
obs_velocity_set_gcs=ones(32,1)*nan;
obs_heading_set_gcs=ones(32,1)*nan;
%传感器的极坐标航向角顺时针为正，世界坐标系下逆时针为正，需要做一个变换
theta_transfer=-obs_theta/180*pi;
%heading方向从正北为0变换为正东为0，同时顺时针和逆时针要变换
heading_transfer=-(obs_heading-90*ones(32,1))/180*pi;

for i=1:32
    if obs_range(i)~=0
        obs_x_set_gcs(i)=host_x+obs_range(i)*cos(host_heading_xy+theta_transfer(i))+3.8*cos(host_heading_xy);%x坐标分为三部分，①车辆的x坐标，②传感器和障碍物在世界坐标系下的x距离，③传感器与车辆坐标原点（后轴中心）的x方向距离
        obs_y_set_gcs(i)=host_y+obs_range(i)*sin(host_heading_xy+theta_transfer(i))+3.8*sin(host_heading_xy);%y坐标的组成与x坐标一致
        obs_velocity_set_gcs(i)=obs_velocity(i);%速度是绝对速度
        obs_heading_set_gcs(i)=heading_transfer(i);%航向角是转换后的航向角
    else
        
    end
    
end

== matlab function testemplanner_cs/Audi_A8_Sedan_1/control module3/control main/lateral control LQR/calc lqr K ==
  data: k1 input; k output; k2 input; k3 input; k4 input; vx input
function k  = fcn(k1,k2,k3,k4,vx)
    if abs(vx)<0.1
        k=[0,0,0,0];
    else
       
        k=[k1,k2,k3,k4];
    end
end

== matlab function testemplanner_cs/Audi_A8_Sedan_1/control module3/control main/lateral control LQR/err_kappa_calculate_module ==
  data: x input; y input; phi input; vx input; vy input; phi_dot input; xr input; yr input; thetar input; kappar input; err output; es output; s_dot output; phi output; projection_point_thetar output
function [err,es,s_dot,phi,projection_point_thetar] = fcn(x,y,phi,vx,vy,phi_dot,xr,yr,thetar,kappar)
    
    tor=[cos(thetar);sin(thetar)];
    nor=[-sin(thetar);cos(thetar)];
    d_err=[x-xr;y-yr];
    ed=nor'*d_err;
    es=tor'*d_err;
    %projection_point_thetar=thetar(dmin);%apollo
    projection_point_thetar=thetar+kappar*es;
    ed_dot=vy*cos(phi-projection_point_thetar)+vx*sin(phi-projection_point_thetar);
    %%%%%%%%%
    ephi=sin(phi-projection_point_thetar);
    %%%%%%%%%
    ss_dot=vx*cos(phi-projection_point_thetar)-vy*sin(phi-projection_point_thetar);
    s_dot=ss_dot/(1-kappar*ed);
    ephi_dot=phi_dot-kappar*s_dot;
    err=[ed;ed_dot;ephi;ephi_dot];
    
    
    
    
    
    
    
    
    
    
    
    


end

== matlab function testemplanner_cs/Audi_A8_Sedan_1/control module3/control main/lateral control LQR/feed_forword_control ==
  data: vx input; a input; forword_angle output; b input; m input; cf input; cr input; k input; kr input
function forword_angle = fcn(vx,a,b,m,cf,cr,k,kr)
    forword_angle=kr*(a+b-b*k(3)-(m*vx*vx/(a+b))*((b/cf)+(a/cr)*k(3)-(a/cr)));
end

== matlab function testemplanner_cs/Audi_A8_Sedan_1/decision&planning module/referenceline provider/MATLAB Function2 ==
  data: path_x input; path_heading output; path_y input; path_kappa output
function [path_heading,path_kappa] = fcn(path_x,path_y)
%%通过全局轨迹点坐标求解轨迹点的航向以及曲率
%输入：坐标点的x,y坐标
%输出：坐标点与x轴夹角航向以及此点的曲率大小
%原理：
%    dheading=atan（dy/dx）
%    dw=dheading/ds
%    ds=sqrt((dx^2+dy^2))
%求航向角时使用atan函数会涉及角的多值性，因此使用四象限atan函数和中点欧拉法求解
dx=diff(path_x);
dy = diff(path_y);
dx_pre=[dx(1);dx];
dx_after=[dx;dx(end)];
dy_pre=[dy(1);dy];
dy_after=[dy;dy(end)];
dx_final=(dx_after+dx_pre)/2;
dy_final=(dy_after+dy_pre)/2;
ds=sqrt(dx_final.^2+dy_final.^2);
d_heading=atan2(dy_final,dx_final);
diff_d_heading=diff(d_heading);
d_heading_pre=[diff_d_heading(1);diff_d_heading];
d_heading_after=[diff_d_heading;diff_d_heading(end)];
d_heading_final=(d_heading_pre+d_heading_after)/2;
dw=sin(d_heading_final)./ds;%使用sin(a)=a,当a非常小时


path_heading=d_heading_final;
path_kappa=dw;
